simulink model "REV3_Harness"  (R2025b)
settings: Solver=ode8  StartTime=0.0  StopTime=inf  FixedStep=0.0001  RelTol=1e-3
settings Model: DataDictionary=rev3_data.sldd  Creator=matat  LastModifiedBy=matat
settings DebuggingCC: ParameterPrecisionLossMsg=none
settings RTWCC: GPUComputeCapability=3.5

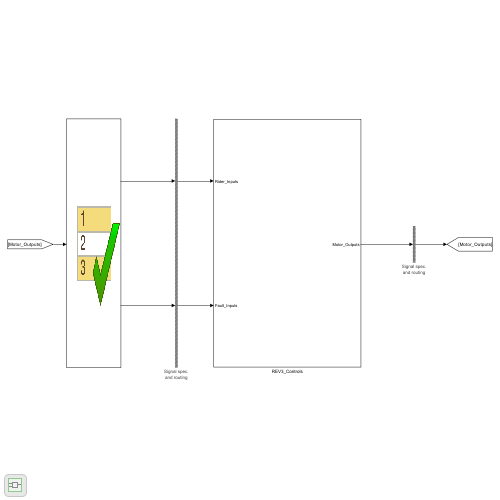
[thumbnail: Simulink's stored preview of the top-level diagram]
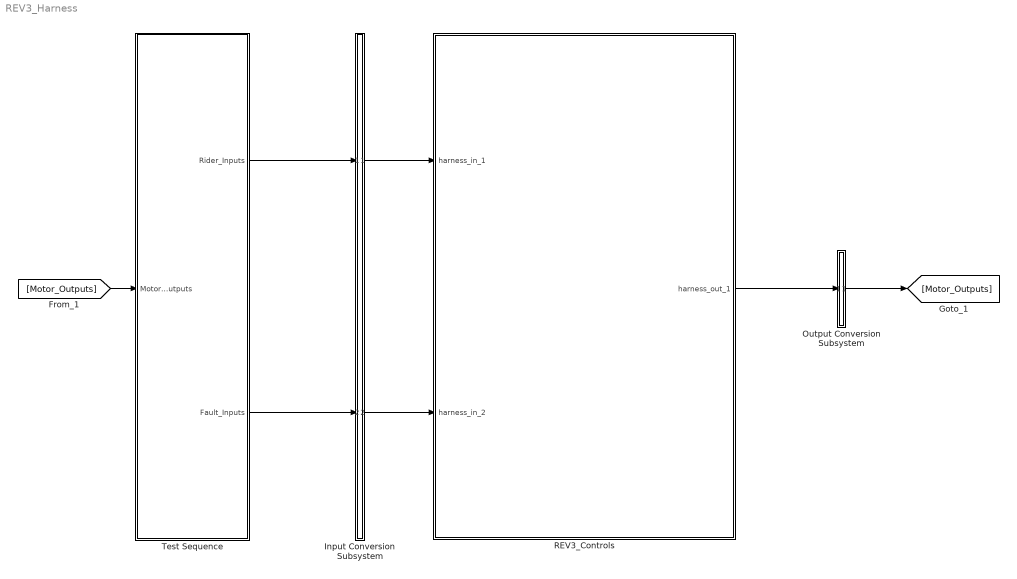
== system REV3_Harness ==
  Input Conversion Subsystem : Subsystem  Tag=__SLT_ICS__  Description=|
      | Signal spec.
      | and routing
      settings: AttributesFormatString=%<Description>
  Output Conversion Subsystem : Subsystem  Tag=__SLT_OCS__  Description=|
      | Signal spec.
      | and routing
      settings: AttributesFormatString=%<Description>
  REV3_Controls : Subsystem  Tag=__SL_testing_harness_stub_
  Test Sequence : Test Sequence  TreatAsAtomicUnit=on
  wires:
  Test Sequence/1(Rider_Inputs) -> Input Conversion Subsystem/1(Inport_1)
  Test Sequence/2(Fault_Inputs) -> Input Conversion Subsystem/2(Inport_2)
  [Motor_Outputs] -> Test Sequence/1(Motor_Outputs)
  Output Conversion Subsystem/1(Outport_1) -> [Motor_Outputs]
  Input Conversion Subsystem/1(Outport_1) -> REV3_Controls/1(harness_in_1)
  Input Conversion Subsystem/2(Outport_2) -> REV3_Controls/2(harness_in_2)
  REV3_Controls/1(harness_out_1) -> Output Conversion Subsystem/1(Inport_1)

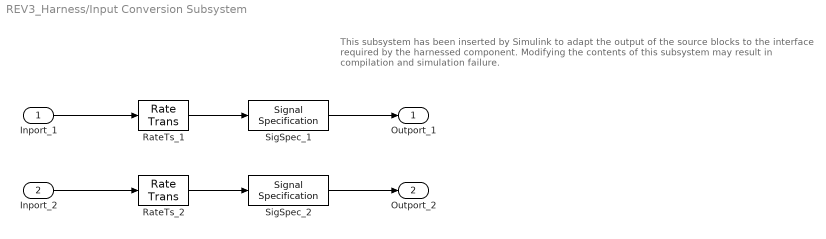
== system REV3_Harness/Input Conversion Subsystem ==
  note: This subsystem has been inserted by Simulink to adapt the output of the source blocks to the interface required by the harnessed component.
      |  Modifying the contents of this subsystem may result in compilation and simulation failure.
  Inport_1 : Inport
  Inport_2 : Inport  Port=2
  RateTs_1 : RateTransition  OutPortSampleTime=0.0001
  RateTs_2 : RateTransition  OutPortSampleTime=0.0001
  SigSpec_1 : SignalSpecification  OutDataTypeStr=Bus: Rider_Inputs  Dimensions=[1]  SampleTime=0.0001  BusOutputAsStruct=on
  SigSpec_2 : SignalSpecification  OutDataTypeStr=Bus: Fault_Inputs  Dimensions=[1]  SampleTime=0.0001  BusOutputAsStruct=on
  Outport_1 : Outport
  Outport_2 : Outport  Port=2
  wires:
  SigSpec_1/1 -> Outport_1/1
  RateTs_1/1 -> SigSpec_1/1
  Inport_1/1 -> RateTs_1/1
  SigSpec_2/1 -> Outport_2/1
  RateTs_2/1 -> SigSpec_2/1
  Inport_2/1 -> RateTs_2/1

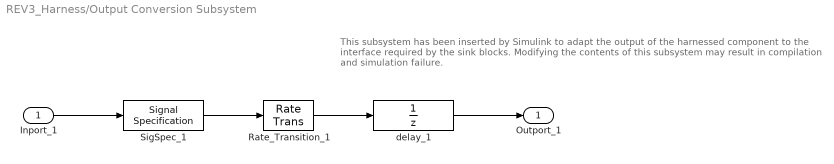
== system REV3_Harness/Output Conversion Subsystem ==
  note: This subsystem has been inserted by Simulink to adapt the output of the harnessed component to the interface required by the sink blocks.
      |  Modifying the contents of this subsystem may result in compilation and simulation failure.
  Inport_1 : Inport
  Rate_Transition_1 : RateTransition  OutPortSampleTimeOpt=Inherit
  SigSpec_1 : SignalSpecification  OutDataTypeStr=Bus: Motor_Outputs  Dimensions=[1]  SampleTime=0.0001  BusOutputAsStruct=on
  delay_1 : UnitDelay  SampleTime=-1
  Outport_1 : Outport
  wires:
  Inport_1/1 -> SigSpec_1/1
  SigSpec_1/1 -> Rate_Transition_1/1
  Rate_Transition_1/1 -> delay_1/1
  delay_1/1 -> Outport_1/1

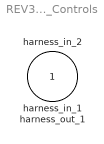
== system REV3_Harness/REV3_Controls ==
  harness_in_1 : Inport
  harness_in_2 : Inport  Port=2
  harness_out_1 : Outport

== stateflow chart REV3_Harness/Test Sequence ==
  settings: updateMethod=DISCRETE  sampleTime=0.0001
  state Run
    %% Initialize data outputs.
    Rider_Inputs.Yes_HIB.Forward_EN = false;
    Rider_Inputs.Yes_HIB.Start = false;
    Rider_Inputs.Yes_HIB.Brake = 0;
    Rider_Inputs.Yes_HIB.Throttle = int16(0);
    Rider_Inputs.No_HIB.Key_In = false;
    Rider_Inputs.No_HIB.Estop_In = false;
    Fault_Inputs.VCU.Override_Ignition = false;
    Fault_Inputs.VCU.Ignition = false;
    Fault_Inputs.VCU.Override_ESTOP = false;
    Fault_Inputs.VCU.ESTOP = false;
    Fault_Inputs.VCU.Override_Brake = false;
    Fault_Inputs.VCU.Brake = false;
    Fault_Inputs.VCU.Override_Forward_EN = false;
    Fault_Inputs.VCU.Forward_EN = false;
    Fault_Inputs.VCU.Override_Start = false;
    Fault_Inputs.VCU.Start = false;
    Fault_Inputs.VCU.Override_Throttle = false;
    Fault_Inputs.VCU.Throttle = 0;
    Fault_Inputs.VCU.Override_HIB_Comparison_Fault = false;
    Fault_Inputs.VCU.HIB_Comparison_Fault = false;
    Fault_Inputs.VCU.Override_Interlock = false;
    Fault_Inputs.VCU.Interlock = false;
    Fault_Inputs.VCU.Override_Inverter_Discharge_State = false;
    Fault_Inputs.VCU.Inverter_Discharge_State = MC_DC_State.Disabled;
    Fault_Inputs.VCU.Override_VSM_State = false;
    Fault_Inputs.VCU.VSM_State = MC_VSM_State.Start;
    Fault_Inputs.VCU.Override_LVSS_ON = false;
    Fault_Inputs.VCU.LVSS_ON = false;
    Fault_Inputs.VCU.Override_Contactor_Closed = false;
    Fault_Inputs.VCU.Contactor_Closed = false;
    Fault_Inputs.VCU.Override_Cell_Temps = false;
    Fault_Inputs.VCU.Cell_Temps = 0;
    Fault_Inputs.VCU.Override_Cell_Voltages = false;
    Fault_Inputs.VCU.Cell_Voltages = 0;
    Fault_Inputs.VCU.Override_Isolation_State = false;
    Fault_Inputs.VCU.Isolation_State = 0;
    Fault_Inputs.VCU.Override_MC_Speed_Out = false;
    Fault_Inputs.VCU.MC_Speed_Out = 0;
    Fault_Inputs.VCU.Override_Batt_Speed_Out = false;
    Fault_Inputs.VCU.Batt_Speed_Out = 0;
    Fault_Inputs.VCU.Override_Temperatures = false;
    Fault_Inputs.VCU.Temperatures = 0;
    Fault_Inputs.VCU.Override_MC_Flow_Rate = false;
    Fault_Inputs.VCU.MC_Flow_Rate = 0;
    Fault_Inputs.VCU.Override_Batt_Flow_Rate = false;
    Fault_Inputs.VCU.Batt_Flow_Rate = 0;
    Fault_Inputs.VCU.Override_HIB_ON = false;
    Fault_Inputs.VCU.HIB_ON = false;
    Fault_Inputs.VCU.Override_HUDL_ON = false;
    Fault_Inputs.VCU.HUDL_ON = false;
    Fault_Inputs.VCU.Override_TMS_ON = false;
    Fault_Inputs.VCU.TMS_ON = false;
    Fault_Inputs.VCU.Override_GUB_ON = false;
    Fault_Inputs.VCU.GUB_ON = false;
    Fault_Inputs.VCU.Override_Acc_ON = false;
    Fault_Inputs.VCU.Acc_ON = false;
    Fault_Inputs.VCU.Override_Batt_12V_ON = false;
    Fault_Inputs.VCU.Batt_12V_ON = false;
    Fault_Inputs.VCU.Override_Vicor_Current = false;
    Fault_Inputs.VCU.Vicor_Current = 0;
    Fault_Inputs.VCU.Override_LVSS_Temps = false;
    Fault_Inputs.VCU.LVSS_Temps = 0;
    Fault_Inputs.VCU.Override_LVSS_Currents = false;
    Fault_Inputs.VCU.LVSS_Currents = 0;
    Fault_Inputs.VCU.Override_Heartbeats = false;
    Fault_Inputs.VCU.Heartbeats = 0;
    Fault_Inputs.VCU.Override_MC_12V0 = false;
    Fault_Inputs.VCU.MC_12V0 = false;
    Fault_Inputs.VCU.Override_LVSS_EN = false;
    Fault_Inputs.VCU.LVSS_EN = false;
    Fault_Inputs.VCU.Override_nReset = false;
    Fault_Inputs.VCU.nReset = false;
    Fault_Inputs.VCU.Override_Self_Test = false;
    Fault_Inputs.VCU.Self_Test = 0;
    Fault_Inputs.VCU.Override_Watchdog = false;
    Fault_Inputs.VCU.Watchdog = false;
    Fault_Inputs.VCU.Override_uC_State = false;
    Fault_Inputs.VCU.uC_State = UC_State.Preset;
    Fault_Inputs.VCU.Override_HB_Feedback = false;
    Fault_Inputs.VCU.HB_Feedback = false;
    Fault_Inputs.VCU.Override_HM_Fault = false;
    Fault_Inputs.VCU.HM_Fault = false;
    Fault_Inputs.VCU.Direction_Command = int16(0);
    Fault_Inputs.VCU.Override_Direction_Command = false;
    Fault_Inputs.VCU.Rolling_Counter = int16(0);
    Fault_Inputs.VCU.Override_Rolling_Counter = false;
    Fault_Inputs.VCU.Speed_Command = int16(0);
    Fault_Inputs.VCU.Override_Speed_Command = false;
    Fault_Inputs.VCU.Speed_Mode_Enable = int16(0);
    Fault_Inputs.VCU.Override_Speed_Mode_Enable = false;
    Fault_Inputs.VCU.Torque_Limit_Command = int16(0);
    Fault_Inputs.VCU.Override_Torque_Limit_Command = false;
    Fault_Inputs.VCU.LS_Self_Test = false;
    Fault_Inputs.VCU.Override_LS_Self_Test = false;
    Fault_Inputs.VCU.MC_Self_Test = false;
    Fault_Inputs.VCU.Override_MC_Self_Test = false;
    Fault_Inputs.VCU.CAN_Self_Test = false;
    Fault_Inputs.VCU.Override_CAN_Self_Test = false;
    Fault_Inputs.VCU.LVSS_EN_Override = false;
    Fault_Inputs.VCU.Override_LVSS_EN_Override = false;
    Fault_Inputs.VCU.MC_EN_Override = false;
    Fault_Inputs.VCU.Override_MC_EN_Override = false;
    Fault_Inputs.VCU.CAN_Override = false;
    Fault_Inputs.VCU.Override_CAN_Override = false;
    Fault_Inputs.BMS.BMS_EN = false;
    Fault_Inputs.BMS.Override_BMS_EN = false;
    Fault_Inputs.BMS.BMS_Contactor_State = BMS_Contactor_Command.Open_Contactor;
    Fault_Inputs.BMS.Override_BMS_Contactor_State = false;
    Fault_Inputs.BMS.BMS_Previous_State = false;
    Fault_Inputs.BMS.Override_BMS_Previous_State = false;
    Fault_Inputs.BMS.Cell_Temps = 0;
    Fault_Inputs.BMS.Override_Cell_Temps = false;
    Fault_Inputs.BMS.Cell_Voltages = 0;
    Fault_Inputs.BMS.Override_Cell_Voltages = false;
    Fault_Inputs.GFDB.GFDB_EN = false;
    Fault_Inputs.GFDB.Override_GFDB_EN = false;
    Fault_Inputs.GFDB.Fault_Value = 0;
    Fault_Inputs.GFDB.Override_Isolation_State = false;
    Fault_Inputs.TMS.TMS_EN = false;
    Fault_Inputs.TMS.Override_TMS_EN = false;
    Fault_Inputs.TMS.MC_Speed = 0;
    Fault_Inputs.TMS.Override_MC_Speed = false;
    Fault_Inputs.TMS.Batt_Speed = 0;
    Fault_Inputs.TMS.Override_Batt_Speed = false;
    Fault_Inputs.TMS.Temperatures = 0;
    Fault_Inputs.TMS.Override_Temperatures = false;
    Fault_Inputs.TMS.Batt_Flow_Rate = 0;
    Fault_Inputs.TMS.Override_Batt_FR = false;
    Fault_Inputs.TMS.MC_Flow_Rate = 0;
    Fault_Inputs.TMS.Override_MC_FR = false;
    Fault_Inputs.HIB.HIB_EN = false;
    Fault_Inputs.HIB.Override_HIB_EN = false;
    Fault_Inputs.HIB.Throttle = 0;
    Fault_Inputs.HIB.Override_Throttle = false;
    Fault_Inputs.HIB.Brake = 0;
    Fault_Inputs.HIB.Override_Brake = false;
    Fault_Inputs.HIB.Start = false;
    Fault_Inputs.HIB.Override_Start = false;
    Fault_Inputs.HIB.Forward_EN = false;
    Fault_Inputs.HIB.Override_Forward_EN = false;
    Fault_Inputs.HIB.Comparison_Error_Count = 0;
    Fault_Inputs.HIB.Override_Comparison_Error_Count = false;
    Fault_Inputs.HIB.Acceptable_Margin_Error_Count = 0;
    Fault_Inputs.HIB.Override_Acceptable_Margin_Error_Count = false;
    Fault_Inputs.HIB.Precision_Margin_Error_Count = 0;
    Fault_Inputs.HIB.Override_Precision_Margin_Error_Count = false;
    Fault_Inputs.LVSS.LVSS_EN = false;
    Fault_Inputs.LVSS.Override_LVSS_EN = false;
    Fault_Inputs.LVSS.TMS_EN = false;
    Fault_Inputs.LVSS.Override_TMS_EN = false;
    Fault_Inputs.LVSS.GUB_EN = false;
    Fault_Inputs.LVSS.Override_GUB_EN = false;
    Fault_Inputs.LVSS.HIB_EN = false;
    Fault_Inputs.LVSS.Override_HIB_EN = false;
    Fault_Inputs.LVSS.HUDL_EN = false;
    Fault_Inputs.LVSS.Override_HUDL_EN = false;
    Fault_Inputs.LVSS.Acc_EN = false;
    Fault_Inputs.LVSS.Override_Acc_EN = false;
    Fault_Inputs.LVSS.Batt_12V_EN = false;
    Fault_Inputs.LVSS.Override_Batt_12V_EN = false;
    Fault_Inputs.LVSS.Vicor_Current = 0;
    Fault_Inputs.LVSS.Override_Vicor_Current = false;
    Fault_Inputs.LVSS.TMS_Temp = 0;
    Fault_Inputs.LVSS.Override_TMS_Temp = false;
    Fault_Inputs.LVSS.TMS_Current = 0;
    Fault_Inputs.LVSS.Override_TMS_Current = false;
    Fault_Inputs.LVSS.HIB_Temp = 0;
    Fault_Inputs.LVSS.Override_HIB_Temp = false;
    Fault_Inputs.LVSS.HIB_Current = 0;
    Fault_Inputs.LVSS.Override_HIB_Current = false;
    Fault_Inputs.LVSS.HUDL_Temp = 0;
    Fault_Inputs.LVSS.Override_HUDL_Temp = false;
    Fault_Inputs.LVSS.HUDL_Current = 0;
    Fault_Inputs.LVSS.Override_HUDL_Current = false;
    Fault_Inputs.LVSS.GUB_Temp = 0;
    Fault_Inputs.LVSS.Override_GUB_Temp = false;
    Fault_Inputs.LVSS.GUB_Current = 0;
    Fault_Inputs.LVSS.Override_GUB_Current = false;
    Fault_Inputs.LVSS.Batt_12V_Temp = 0;
    Fault_Inputs.LVSS.Override_Batt_12V_Temp = false;
    Fault_Inputs.LVSS.Batt_12V_Current = 0;
    Fault_Inputs.LVSS.Override_Batt_12V_Current = false;
    Fault_Inputs.LVSS.Acc_Temp = 0;
    Fault_Inputs.LVSS.Override_Acc_Temp = false;
    Fault_Inputs.LVSS.Acc_Current = 0;
    Fault_Inputs.LVSS.Override_Acc_Current = false;
    Fault_Inputs.LVSS.LVSS_Currents = 0;
    Fault_Inputs.LVSS.Override_LVSS_Currents = false;
    Fault_Inputs.LVSS.LVSS_Temps = 0;
    Fault_Inputs.LVSS.Override_LVSS_Temps = false;
  (default) -> Run
  data: Motor_Outputs input Bus: Motor_Outputs size=[1]; Rider_Inputs output Bus: Rider_Inputs size=[1]; Fault_Inputs output Bus: Fault_Inputs size=[1]
